simulink model "plant_obscon_filter"  (Simulink 7.9)
settings: Solver=ode45  StartTime=0.0  StopTime=40  RelTol=1e-3
values from neighbouring files (symbols this model uses):
  A = [1 2 0; 3 1 -2; 4 -2 1]    [calcul_gains.m]    (also in script.m; script1.m)
  Aa = [A Bd; 0 0 0 0]    [calcul_gains.m]    (also in script.m; script1.m)
  B = [1; -1; 1]    [calcul_gains.m]    (also in script.m; script1.m)
  Ba = [B; 0]    [calcul_gains.m]    (also in script.m; script1.m)
  Bd = [0; 1; 0]    [calcul_gains.m]    (also in script.m; script1.m)
  C = [7 8 1]    [calcul_gains.m]    (also in script.m; script1.m)
  Ca = [C 0]    [calcul_gains.m]    (also in script.m; script1.m)
  D = 0    [calcul_gains.m]    (also in script.m; script1.m)
  dbar = 0    [script.m]    (also in script1.m)
  Dd = 0    [calcul_gains.m]    (also in script.m; script1.m)
  k = -1/(C*inv(A-B*K)*B)    [script.m]    (also in script1.m)
  K = place(A,B,vpc)    [script.m]    (also in script1.m)
  kd = C*inv(A-B*K)*Bd/(C*inv(A-B*K)*B)    [script.m]    (also in script1.m)
  La = La'    [calcul_gains.m]    (also in script.m = transpose(place(Aa',Ca',vpo)); script1.m = transpose(place(Aa',Ca',vpo)))
  ubar = xubar(4)    [script.m]    (also in script1.m)
  xaestbar = [0; 0; 0; 0]    [script.m]    (also in script1.m)
  xbar = xubar(1:3)    [script.m]    (also in script1.m)
  ybar = -2    [script.m]    (also in script1.m)
libraries: cstblocks x1, simulink x1
settings Model: Creator=PhM  LastModifiedBy=PhM
settings OptimizationCC: InitFltsAndDblsToZero=on
settings DebuggingCC: SaveWithParameterizedLinksMsg=none  SignalResolutionControl=TryResolveAllWithWarning  MultiTaskDSMMsg=warning  MultiTaskCondExecSysMsg=none  FcnCallInpInsideContextMsg=Use local settings  StrictBusMsg=None
settings RTWCC: IncludeERTFirstTime=on
settings GRTTargetCC: TargetFcnLib=ansi_tfl_tmw.mat  CombineOutputUpdateFcns=off  GRTInterface=on

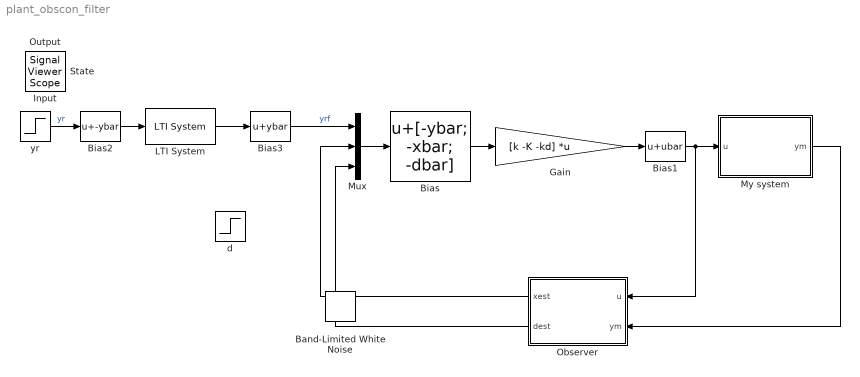
== system plant_obscon_filter ==
  Bias : Bias  Bias=[-ybar; -xbar; -dbar]
  Bias1 : Bias  Bias=ubar
  Bias2 : Bias  Bias=-ybar
  Bias3 : Bias  Bias=ybar
  Gain : Gain  Gain=[k -K -kd]  Multiplication=Matrix(K*u) (u vector)
  LTI System : cstblocks/LTI System  sys=sysf  IC=[]
  Mux : Mux  Inputs="[1 3  1]"
  My system : Subsystem
  Observer : Subsystem
  yr : Step  Time=5  Before=ybar  After=ybar+1  SampleTime=0
  Band-Limited White Noise : simulink/Sources/Band-Limited White Noise  IOType=siggen  Cov=1e-6*0  Ts=1e-2  seed=[23341]
  Input : SignalViewerScope  IOType=viewer  NumInputPorts=2  LegendLocations="0.72634     0.90138     0.19753    0.035179 0.65535      0.4158     0.26852    0.062284"  RefreshTime=0.035000
      settings: ShowLegends=on  TimeRange=40  YMin=-0.4~-0.0025  YMax=0.45~0.05  SaveName=ScopeData2
  Output : SignalViewerScope  IOType=viewer  NumInputPorts=2  RefreshTime=0.035000
      settings: TimeRange=40  YMin=-2~-2  YMax=2.25~2.25
  State : SignalViewerScope  IOType=viewer  ZoomMode=yonly  RefreshTime=0.035000
      settings: TimeRange=40  YMin=-0.4  YMax=0.45
  d : Step  IOType=siggen  Time=10  Before=dbar  After=dbar+0.05  SampleTime=0
  wires:
  My system/1(ym) -> Observer/2(ym)
  Gain/1 -> Bias1/1
  Mux/1 -> Bias/1
  Bias/1 -> Gain/1
  Bias1/1 -> My system/1(u), Observer/1(u)
  yr/1 -> Bias2/1  "yr"
  Observer/1(xest) -> Mux/2
  Observer/2(dest) -> Mux/3
  LTI System/1 -> Bias3/1
  Bias2/1 -> LTI System/1
  Bias3/1 -> Mux/1  "yrf"

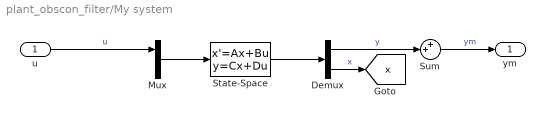
== system plant_obscon_filter/My system ==
  u : Inport
  Demux : Demux  Outputs=[1 3]
  Mux : Mux  Inputs=2
  State-Space : StateSpace  A=A  B=[B Bd]  C=[C; eye(3)]  D=[D Dd; zeros(3,2)]  X0=xbar
  Sum : Sum  Inputs=++|
  ym : Outport
  tag scope: x=global
  wires:
  Mux/1 -> State-Space/1
  State-Space/1 -> Demux/1
  Demux/1 -> Sum/2  "y"
  Demux/2 -> [x]  "x"
  u/1 -> Mux/1  "u"
  Sum/1 -> ym/1  "ym"

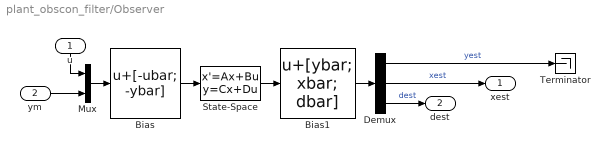
== system plant_obscon_filter/Observer ==
  u : Inport
  ym : Inport  Port=2
  Bias : Bias  Bias=[-ubar; -ybar]
  Bias1 : Bias  Bias=[ybar; xbar; dbar]
  Demux : Demux  Outputs=[1 3 1]
  Mux : Mux  Inputs=2
  State-Space : StateSpace  A=Aa-La*Ca  B=[Ba La]  C=[Ca; eye(4)]  D=zeros(5,2)  X0=xaestbar
  Terminator : Terminator
  xest : Outport
  dest : Outport  Port=2
  wires:
  Mux/1 -> Bias/1
  State-Space/1 -> Bias1/1
  u/1 -> Mux/1
  ym/1 -> Mux/2
  Demux/1 -> Terminator/1  "yest"
  Demux/2 -> xest/1  "xest"
  Demux/3 -> dest/1  "dest"
  Bias/1 -> State-Space/1
  Bias1/1 -> Demux/1
